simulink model "simple_model"  (R2018a)
settings: Solver=VariableStepAuto  StartTime=0.0  StopTime=10.0  RelTol=1e-3
settings Model: Creator=careerist  LastModifiedBy=careerist

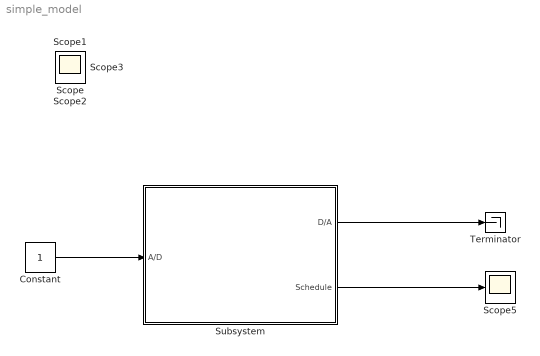
== system simple_model ==
  Constant : Constant
  Scope{,1..3,5} (5 alike) : Scope
  Subsystem : Subsystem  mask{sfunc='sched_init', args='RoundRobin', in_out_vec=[1 2]}
      mask prompts: sfunc "Name of init func"; args "init func arguments"; in_out_vec "input and output ports"
      mask init:
      | init_kernel(gcb,{sfunc,args,in_out_vec})
      settings: MinAlgLoopOccurrences=on
      mask Display:
      | color('red');
      | text(0.35,0.5,'X-KERNEL')
  Terminator : Terminator
  wires:
  Constant/1 -> Subsystem/1(A/D)
  Subsystem/1(D/A) -> Terminator/1
  Subsystem/2(Schedule) -> Scope5/1

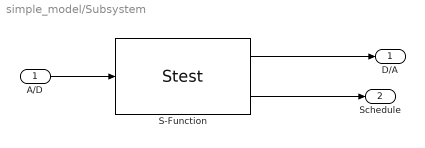
== system simple_model/Subsystem ==
  A/D : Inport
  S-Function : S-Function  FunctionName=Stest  Parameters=sfunc,args,in_out_vec  SFunctionDeploymentMode=off  EnableBusSupport=off
  D/A : Outport
  Schedule : Outport  Port=2
  wires:
  A/D/1 -> S-Function/1
  S-Function/1 -> D/A/1
  S-Function/2 -> Schedule/1
